simulink model "DSimulator_robot3GDL"  (Simulink 10.3)
settings: Solver=ode1  StartTime=0  StopTime=50  FixedStep=0.004  RelTol=1e-3  EnableMultiTasking=on
undefined symbols (not defined in the file or in its folder): Dinamic_ur10_3DOF, SimpleRobotPlotROS, Tau, TrajGen
libraries: simulink x6
settings Model: Creator=E. Dean  LastModifiedBy=gin  MultithreadedSim=on
settings SolverCC: AlgebraicLoopSolver=Auto
settings DataIOCC: LimitDataPoints=on
settings DebuggingCC: SolverPrmCheckMsg=warning  AllowSymbolicDim=off
settings ConfigComp: CovSFcnEnable=off

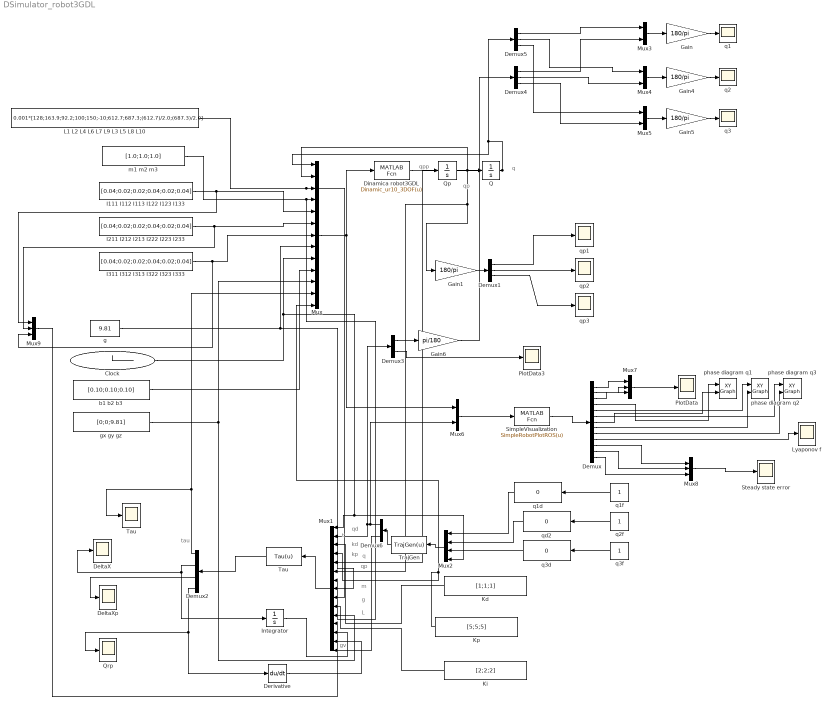
== system DSimulator_robot3GDL ==
  note: gv
  note: qd
  note: q
  note: qp
  note: qpp
  note: tau
  note: t
  note: L
  note: g
  note: m
  note: kp
  note: kd
  note: qp
  note: q
  Clock : Clock
  DeltaX : Scope
  DeltaXp : Scope
  Demux : Demux  Outputs=13
  Demux1 : Demux  Outputs=3
  Demux2 : Demux
  Demux3 : Demux  Outputs=2
  Demux4 : Demux  Outputs=3
  Demux5 : Demux  Outputs=3
  Demux6 : Demux  Outputs=[6;1]
  Derivative : Derivative
  Dinamica robot3GDL : MATLABFcn  MATLABFcn=Dinamic_ur10_3DOF(u)  OutputDimensions=3
  Gain{,1,4..5} (4 alike) : Gain  Gain=180/pi
  Gain6 : Gain  Gain=pi/180
  I111 I112 I113 I122 I123 I133 : Constant  Value=[0.04;0.02;0.02;0.04;0.02;0.04]
  I211 I212 I213 I222 I223 I233 : Constant  Value=[0.04;0.02;0.02;0.04;0.02;0.04]
  I311 I312 I313 I322 I323 I333 : Constant  Value=[0.04;0.02;0.02;0.04;0.02;0.04]
  Integrator : Integrator  InitialCondition=[0.0;0.0;0.0]
  "Kd " : Constant  Value=[1;1;1]
  Ki : Constant  Value=[2;2;2]
  Kp : Constant  Value=[5;5;5]
  "L1 L2 L4 L6 L7 L9 L3 L5 L8 L10 " : Constant  Value=0.001*[128;163.9;92.2;100;150;-10;612.7;687.3;(612.7)/2.0;(687.3)/2.0]
  Lyaponov f : Scope
  Mux : Mux  Inputs=13
  Mux1 : Mux  Inputs=15
  Mux2 : Mux
  Mux{3..6} (4 alike) : Mux  Inputs=2
  Mux7 : Mux  Inputs=3
  Mux8 : Mux  Inputs=3
  Mux9 : Mux  Inputs=3
  PlotData : Scope
  PlotData3 : Scope
  Q : Integrator  InitialCondition=[0;-pi/2;pi/2]
  Qp : Integrator  InitialCondition=[0;0;0]
  Qrp : Scope
  SimpleVisualization : MATLABFcn  MATLABFcn=SimpleRobotPlotROS(u)  OutputDimensions=13
  Steady state error : Scope
  Tau : Scope
  "Tau " : MATLABFcn  MATLABFcn=Tau(u)  OutputDimensions=12  OutputSignalType=real
  TrajGen : MATLABFcn  MATLABFcn=TrajGen(u)  OutputDimensions=7
  "b1 b2 b3 " : Constant  Value=[0.10;0.10;0.10]
  g : Constant  Value=9.81
  gx gy gz : Constant  Value=[0;0;9.81]
  "m1 m2 m3 " : Constant  Value=[1.0;1.0;1.0]
  phase diagram q1 : simulink/Sinks/XY Graph  xmin=-10  xmax=10  ymin=-10  ymax=10  st=-1
  phase diagram q2 : simulink/Sinks/XY Graph  xmin=-10  xmax=10  ymin=-10  ymax=10  st=-1
  phase diagram q3 : simulink/Sinks/XY Graph  xmin=-10  xmax=10  ymin=-10  ymax=10  st=-1
  q1 : Scope
  q1d : simulink/Math Operations/Slider Gain  gain=0  low=-180  high=180
  q1f : Constant
  q2 : Scope
  q2f : Constant
  q3 : Scope
  q3d : simulink/Math Operations/Slider Gain  gain=0  low=-180  high=180
  q3f : Constant
  qd2 : simulink/Math Operations/Slider Gain  gain=0  low=-180  high=180
  qp1 : Scope
  qp2 : Scope
  qp3 : Scope
  wires:
  Dinamica robot3GDL/1 -> Qp/1
  Gain/1 -> q1/1
  Gain1/1 -> Demux1/1
  Demux1/1 -> qp1/1
  Demux1/2 -> qp2/1
  Demux1/3 -> qp3/1
  I111 I112 I113 I122 I123 I133/1 -> Mux9/1, Mux/5
  I211 I212 I213 I222 I223 I233/1 -> Mux9/2, Mux/6
  I311 I312 I313 I322 I323 I333/1 -> Mux9/3, Mux/7
  "b1 b2 b3 "/1 -> Mux/10
  Mux/1 -> Mux6/1, Dinamica robot3GDL/1
  Mux1/1 -> "Tau "/1
  q1f/1 -> q1d/1
  q2f/1 -> qd2/1
  q3f/1 -> q3d/1
  Mux2/1 -> TrajGen/1
  q1d/1 -> Mux2/1
  qd2/1 -> Mux2/2
  q3d/1 -> Mux2/3
  "Kd "/1 -> Mux1/3
  Kp/1 -> Mux1/4, Mux/13
  Q/1 -> Demux5/1, Mux/1, Mux1/5
  Qp/1 -> Q/1, Mux1/6, Gain1/1, Mux/2
  "Tau "/1 -> Demux2/1
  "m1 m2 m3 "/1 -> Mux1/7, Mux/4
  g/1 -> Mux1/8, Mux/8
  "L1 L2 L4 L6 L7 L9 L3 L5 L8 L10 "/1 -> Mux1/9, Mux/3
  Clock/1 -> Mux2/4, Mux1/1, Mux/9
  Ki/1 -> Mux1/10
  Demux3/1 -> Gain6/1
  Demux4/1 -> Mux3/2
  Mux3/1 -> Gain/1
  Gain4/1 -> q2/1
  Mux4/1 -> Gain4/1
  Gain5/1 -> q3/1
  Mux5/1 -> Gain5/1
  Demux5/1 -> Mux3/1
  Demux5/2 -> Mux4/1
  Gain6/1 -> Demux4/1
  Mux6/1 -> SimpleVisualization/1
  Demux2/1 -> Tau/1, Mux/12
  gx gy gz/1 -> Mux1/11, Mux/11
  Demux5/3 -> Mux5/1
  Demux4/2 -> Mux4/2
  Demux4/3 -> Mux5/2
  Demux3/2 -> PlotData3/1
  SimpleVisualization/1 -> Demux/1
  Demux/1 -> Mux7/1
  Demux/2 -> Mux7/2
  Demux/3 -> Mux7/3
  Mux7/1 -> PlotData/1
  Demux/4 -> phase diagram q1/1
  Demux/5 -> phase diagram q2/1
  Demux/6 -> phase diagram q3/1
  Demux/7 -> phase diagram q1/2
  Demux/8 -> phase diagram q2/2
  Demux/9 -> phase diagram q3/2
  Demux/10 -> Lyaponov f/1
  Demux/11 -> Mux8/1
  Demux/12 -> Mux8/2
  Demux/13 -> Mux8/3
  Mux8/1 -> Steady state error/1
  Demux2/3 -> DeltaXp/1
  Demux2/2 -> DeltaX/1, Integrator/1
  Mux9/1 -> Mux1/12
  Integrator/1 -> Mux1/13
  Derivative/1 -> Mux1/14
  Demux2/4 -> Qrp/1, Derivative/1
  Demux6/1 -> Mux6/2, Demux3/1, Mux1/2
  Demux6/2 -> Mux1/15
  TrajGen/1 -> Demux6/1
